simulink model "BPSKImageTransfer"  (R2016a)
settings: Solver=VariableStepDiscrete  SolverMode=SingleTasking  StartTime=0.0  StopTime=420800  RelTol=1e-3
libraries: commlibv2 x8, commutil2 x2, commcnvcod2 x2, commdigbbndpm3 x2, commchan3 x1, commhdledac x1, commhdllib x1, commdigbbnd2 x1
settings Model: Creator=Glynis  LastModifiedBy=Glynis
settings DataIOCC: LimitDataPoints=on  SaveOutput=off  SaveTime=off
settings OptimizationCC: BooleanDataType=off  DefaultParameterBehavior=Inlined  LocalBlockOutputs=off
settings DebuggingCC: AlgebraicLoopMsg=error  SingleTaskRateTransMsg=error  AllowSymbolicDim=off
settings ConfigComp: CovModelRefEnable=Off  CovSFcnEnable=off

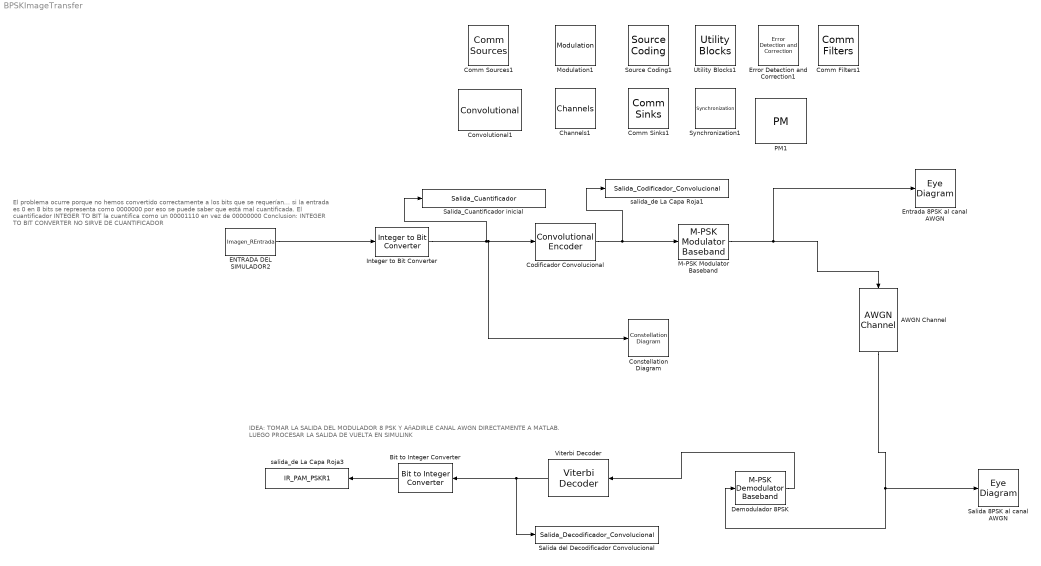
== system BPSKImageTransfer ==
  note: El problema ocurre porque no hemos convertido correctamente a los bits que se requerían...
      | si la entrada es 0 en 8 bits se representa como 0000000 por eso se puede saber que
      | está mal cuantificada.
      |
      | El cuantificador INTEGER TO BIT la cuantifica como un
      | 00001110
      | en vez de
      | 00000000
      |
      | Conclusion: INTEGER TO BIT CONVERTER NO SIRVE DE CUANTIFICADOR
  note: IDEA: TOMAR LA SALIDA DEL MODULADOR 8 PSK Y AñADIRLE CANAL AWGN DIRECTAMENTE A MATLAB. LUEGO PROCESAR LA SALIDA DE VUELTA EN SIMULINK
  AWGN Channel : commchan3/AWGN Channel  InputProcessing=Columns as channels (frame based)  seed=654  noiseMode="Signal to noise ratio  (Eb/No)"  EbNodB=100  EsNodB=10  SNRdB=10  bitsPerSym=8  Ps=1000  Tsym=1  variance=1
  Bit to Integer Converter : commutil2/Bit to Integer Converter  nbits=8  bitOrder=MSB first  signedOutputValues=Unsigned  outDtype=double  outDtypeSigned=Inherit via internal rule
  Channels1 : commlibv2/Channels
  Codificador Convolucional : commcnvcod2/Convolutional Encoder  trellis=poly2trellis(7, [171 133])  opMode=Truncated (reset every frame)  DelayedResetAction=on  hasIniStPort=off  hasFinStPort=off  usePuncVector=off  punctureVector=[1; 1; 0; 1; 0; 1]  reset=Unused parameter value
  Comm Filters1 : commlibv2/Comm Filters
  Comm Sinks1 : commlibv2/Comm Sinks
  Comm Sources1 : commlibv2/Comm Sources
  Constellation Diagram : ConstellationDiagram
  Convolutional1 : commhdledac/Convolutional
  Demodulador 8PSK : commdigbbndpm3/M-PSK Demodulator Baseband  M=8  OutType=Integer  DecType=Hard decision  VarSource=Dialog  Variance=1  Dec=Gray  Mapping=[0:7]  Ph=pi/8  outDtype1=Inherit via internal rule  outDtype2=Inherit via internal rule  derotateFactorWordLen=16  derotateFactorDataTypeStr=Inherit: Same word length as input  derotateFactorLastDataTypeStr=Inherit: Same word length as input
  ENTRADA DEL SIMULADOR2 : FromWorkspace  VariableName=Imagen_REntrada  SampleTime=1  OutputAfterFinalValue=Holding final value
  Entrada 8PSK al canal AWGN : EyeDiagram
  Error Detection and Correction1 : commhdllib/Error Detection and Correction
  Integer to Bit Converter : commutil2/Integer to Bit Converter  nbits=8  signedInputValues=Unsigned  bitOrder=MSB first  outDtype=double
  M-PSK Modulator Baseband : commdigbbndpm3/M-PSK Modulator Baseband  M=8  InType=Integer  Enc=Gray  Mapping=[0:7]  Ph=pi/8  outDtype=double  outWordLen=16  outUDDataType=sfix(16)  outFracLenMode=Best precision  outFracLen=15  outDataTypeStr=double  outLastDataTypeStr=double
  Modulation1 : commlibv2/Modulation
  PM1 : commdigbbnd2/PM
  Salida 8PSK al canal AWGN : EyeDiagram
  "Salida del Decodificador Convolucional " : ToWorkspace  VariableName=Salida_Decodificador_Convolucional  SampleTime=-1
      settings: Save2DSignal=2-D array (concatenate along first dimension)
  "Salida_Cuantificador inicial " : ToWorkspace  VariableName=Salida_Cuantificador  SampleTime=-1
      settings: Save2DSignal=2-D array (concatenate along first dimension)
  Source Coding1 : commlibv2/Source Coding
  Synchronization1 : commlibv2/Synchronization
  Utility Blocks1 : commlibv2/Utility Blocks
  Viterbi Decoder : commcnvcod2/Viterbi Decoder  trellis=poly2trellis(7, [171 133])  isPunctured=off  punctureVector=[1; 1; 0; 1; 0; 1]  erasures=off  dectype=Hard decision  nsdecb=4  runSigValErrCheck=off  tbdepth=34  opmode=Continuous  reset=off  delayedResetAction=on  smWordLength=16  outDataType=Smallest unsigned integer
  salida_de La Capa Roja1 : ToWorkspace  VariableName=Salida_Codificador_Convolucional  SampleTime=-1
      settings: Save2DSignal=2-D array (concatenate along first dimension)
  salida_de La Capa Roja3 : ToWorkspace  VariableName=IR_PAM_PSKR1  SampleTime=1
      settings: Save2DSignal=2-D array (concatenate along first dimension)
  wires:
  Demodulador 8PSK/1 -> Viterbi Decoder/1
  AWGN Channel/1 -> Salida 8PSK al canal AWGN/1, Demodulador 8PSK/1
  M-PSK Modulator Baseband/1 -> Entrada 8PSK al canal AWGN/1, AWGN Channel/1
  Codificador Convolucional/1 -> M-PSK Modulator Baseband/1, salida_de La Capa Roja1/1
  Integer to Bit Converter/1 -> "Salida_Cuantificador inicial "/1, Constellation Diagram/1, Codificador Convolucional/1
  Viterbi Decoder/1 -> "Salida del Decodificador Convolucional "/1, Bit to Integer Converter/1
  Bit to Integer Converter/1 -> salida_de La Capa Roja3/1
  ENTRADA DEL SIMULADOR2/1 -> Integer to Bit Converter/1
